simulink model "Bi_DAB"  (R2023a)
settings: Solver=ode23tb  StartTime=0.0  StopTime=0.1  MaxStep=1e-7  RelTol=1e-7
model workspace (MAT data in the model file):
  Ki = 0.0018
  Kp = 0.05
libraries: spsMosfetLib x8, spsSeriesRLCBranchLib x5, spsCurrentMeasurementLib x4, spsVoltageMeasurementLib x4, spsDCVoltageSourceLib x1, spsLinearTransformerLib x1, slpidlib x1, sps_lib x1
settings Model: Creator=gaming3  LastModifiedBy=gaming3

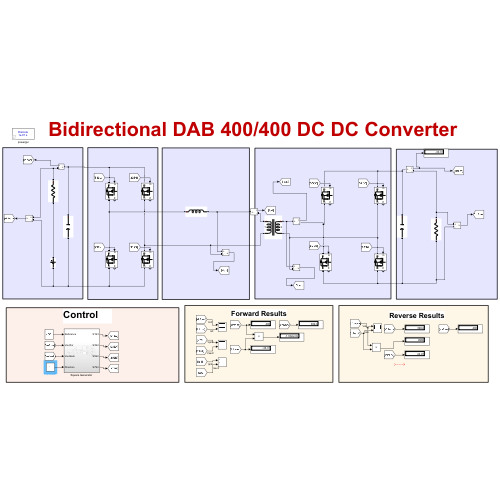
[thumbnail: Simulink's stored preview of the top-level diagram]
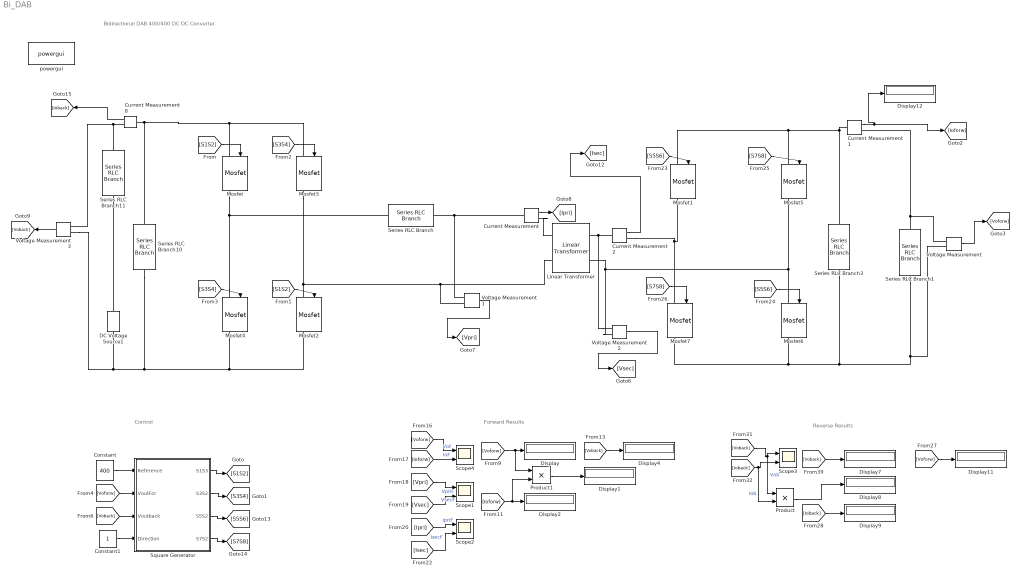
== system Bi_DAB ==
  note: Control
  note: Forward Results
  note: Reverse Results
  note: Bidirectional DAB 400/400 DC DC Converter
  Constant : Constant  Value=400
  Constant1 : Constant
  Current Measurement{,1..2,8} (4 alike) : spsCurrentMeasurementLib/Current Measurement  PhasorSimulation=off  OutputType=Complex  PSBequivalent=0
  DC Voltage Source1 : spsDCVoltageSourceLib/DC Voltage Source  Amplitude=400  Measurements=None
  Display{,1..2,4,7..9,11..12} (9 alike) : Display
  Linear Transformer : spsLinearTransformerLib/Linear Transformer  UNITS=SI  NominalPower=[ 10e3 100e3 ]  winding1=[400 0 0]  winding2=[400 0 0]  ThreeWindings=off  winding3=[3.15e+05 1.9845e+05 12.634]  RmLm=[1.0804e+06 0]  Measurements=None  DataType=on
  Mosfet{,1..7} (8 alike) : spsMosfetLib/Mosfet  Ron=0.1  Lon=0  Rd=0.01  Vfd=0  IC=0  Rs=1e5  Cs=inf  Measurements=on
  Product : Product
  Product1 : Product
  Scope{1..4} (4 alike) : Scope  NumInputPorts=2
  Series RLC Branch : spsSeriesRLCBranchLib/Series RLC Branch  LConnTagsString=__new0  RConnTagsString=__new0  BranchType=L  Resistance=1  Inductance=1.5e-5  SetiL0=off  InitialCurrent=0  Capacitance=1e-6  Setx0=off  InitialVoltage=0  Measurements=None
  Series RLC Branch1 : spsSeriesRLCBranchLib/Series RLC Branch  LConnTagsString=__new0  RConnTagsString=__new0  BranchType=R  Resistance=16  Inductance=1e-3  SetiL0=off  InitialCurrent=0  Capacitance=500e-6  Setx0=on  InitialVoltage=100  Measurements=None
  Series RLC Branch10 : spsSeriesRLCBranchLib/Series RLC Branch  LConnTagsString=__new0  RConnTagsString=__new0  BranchType=C  Resistance=1  Inductance=1e-3  SetiL0=off  InitialCurrent=0  Capacitance=100e-6  Setx0=on  InitialVoltage=400  Measurements=None
  Series RLC Branch11 : spsSeriesRLCBranchLib/Series RLC Branch  LConnTagsString=__new0  RConnTagsString=__new0  BranchType=R  Resistance=0.001  Inductance=1e-3  SetiL0=off  InitialCurrent=0  Capacitance=500e-6  Setx0=on  InitialVoltage=100  Measurements=None
  Series RLC Branch3 : spsSeriesRLCBranchLib/Series RLC Branch  LConnTagsString=__new0  RConnTagsString=__new0  BranchType=C  Resistance=1  Inductance=1e-3  SetiL0=off  InitialCurrent=0  Capacitance=100e-6  Setx0=on  InitialVoltage=400  Measurements=None
  "Square Generator " : Subsystem
  Voltage Measurement{,1..3} (4 alike) : spsVoltageMeasurementLib/Voltage Measurement  PhasorSimulation=off  OutputType=Complex  PSBequivalent=0
  powergui : sps_lib/powergui  Priority=1  SimulationMode=Discrete  SampleTime=1e-07  frequency=60  Iterations=50  frequencyindice=0  Pbase=100e6  ErrMax=1e-4  UnitsV=kV  UnitsW=MW  buscounter=0  FunctionMessages=off  echomessages=off  EnableUseOfTLC=off  CurrentSourceSwitches=off  DisableSnubberDevices=off  DisableRonSwitches=off  DisableVfSwitches=off  DisplayEquations=off  AutomaticDiscreteSolvers=off  SolverType=Tustin/Backward Euler (TBE)  Interpol=off  ExternalGateDelay=off  methode=off  Ts=100  x0status=blocks  SPID=on  SwTol=0  HookPort=off  NonlinearTolerance=1e-4  nMaxIteration=100  ContinueOnMaxIteration=off  RestoreLinks=warning  ResistiveCurrentMeasurement=off  Frange=[0:2:500]  Ylog=off  Xlog=on  ShowGrid=off  save=off  variable=ZData  structure=0  ZoomFFT=off  StartTime=0.0  cycles=1  DisplayStyle=1  fundamental=60  FreqAxis=off  MaxFrequency=1000  frequencyindicesteady=1  RmsSteady=1  display=off
  wires:
  Current Measurement/1 -> [Ipri]
  Current Measurement1/1 -> [Ioforw], Display12/1
  Voltage Measurement1/1 -> [Vpri]
  Current Measurement8/1 -> [Ioback]
  Voltage Measurement3/1 -> [Voback]
  Voltage Measurement2/1 -> [Vsec]
  Current Measurement2/1 -> [Isec]
  "Square Generator "/2(S3S2) -> [S3S4]
  "Square Generator "/4(S7S2) -> [S7S8]
  Constant1/1 -> "Square Generator "/4(Direction)
  "Square Generator "/1(S1S3) -> [S1S2]
  [Voforw] -> "Square Generator "/2(VoutFor)
  Constant/1 -> "Square Generator "/1(Reference)
  "Square Generator "/3(S5S2) -> [S5S6]
  [Ioforw] -> Product1/2, Display2/1
  [Ioforw] -> Scope4/2  "IoF"
  [Isec] -> Scope2/2  "IsecF"
  [Vpri] -> Scope1/1  "VpriF"
  [Voforw] -> Scope4/1  "VoF"
  [Voback] -> Display4/1
  [Voback] -> Display7/1
  [Voforw] -> Display11/1
  [Ipri] -> Scope2/1  "IpriF"
  [Voback] -> Scope3/1, Product/1  "Vob"
  [Voforw] -> Product1/1, Display/1
  [Ioback] -> Display9/1
  Product/1 -> Display8/1
  ? -> ?
  [Ioback] -> Scope3/2, Product/2  "Iob"
  [Vsec] -> Scope1/2  "VsecF"
  [S1S2] -> Mosfet/1
  [S3S4] -> Mosfet3/1
  [S1S2] -> Mosfet2/1
  [S3S4] -> Mosfet4/1
  [S7S8] -> Mosfet7/1
  [S5S6] -> Mosfet6/1
  [S7S8] -> Mosfet5/1
  [S5S6] -> Mosfet1/1
  [Voback] -> "Square Generator "/3(Voutback)
  Voltage Measurement/1 -> [Voforw]
  Product1/1 -> Display1/1
  connections:
  Current Measurement8/RConn1 -- Series RLC Branch11/LConn1 -- Voltage Measurement3/LConn1
  Mosfet1/RConn1 -- Current Measurement2/RConn1 -- Mosfet7/LConn1
  Mosfet5/LConn1 -- Series RLC Branch3/LConn1 -- Current Measurement1/LConn1 -- Mosfet1/LConn1
  Voltage Measurement1/LConn1 -- Current Measurement/LConn1 -- Series RLC Branch/RConn1
  Mosfet3/RConn1 -- Linear Transformer/LConn2 -- Voltage Measurement1/LConn2 -- Mosfet2/LConn1
  Mosfet2/RConn1 -- Series RLC Branch10/RConn1 -- Voltage Measurement3/LConn2 -- DC Voltage Source1/LConn1 -- Mosfet4/RConn1
  Current Measurement8/LConn1 -- Mosfet/LConn1 -- Mosfet3/LConn1 -- Series RLC Branch10/LConn1
  Mosfet5/RConn1 -- Mosfet6/LConn1 -- Linear Transformer/RConn2 -- Voltage Measurement2/LConn2
  Mosfet7/RConn1 -- Series RLC Branch3/RConn1 -- Series RLC Branch1/RConn1 -- Voltage Measurement/LConn2 -- Mosfet6/RConn1
  Voltage Measurement2/LConn1 -- Current Measurement2/LConn1 -- Linear Transformer/RConn1
  Mosfet4/LConn1 -- Series RLC Branch/LConn1 -- Mosfet/RConn1
  Current Measurement/RConn1 -- Linear Transformer/LConn1
  Series RLC Branch1/LConn1 -- Current Measurement1/RConn1 -- Voltage Measurement/LConn1
  Series RLC Branch11/RConn1 -- DC Voltage Source1/RConn1

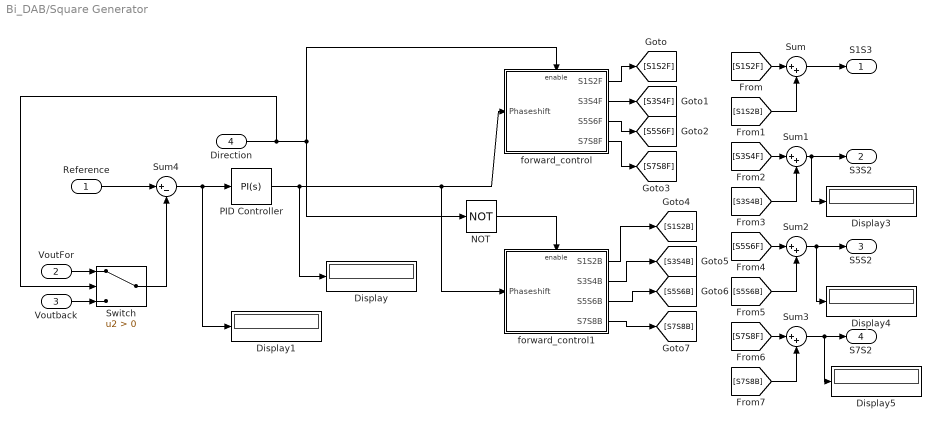
== system Bi_DAB/Square Generator  ==
  Reference : Inport
  VoutFor : Inport  Port=2
  Voutback : Inport  Port=3
  Direction : Inport  Port=4
  Display{,1,3..5} (5 alike) : Display
  NOT : Logic  Operator=NOT  IconShape=distinctive  AllPortsSameDT=off  OutDataTypeStr=boolean
  PID Controller : slpidlib/PID Controller  Controller=PI  Form=Parallel  TimeDomain=Continuous-time  UseExternalTs=off  SampleTime=-1  IntegratorMethod=Forward Euler  FilterMethod=Forward Euler  ControllerParametersSource=internal  P=0.000085  I=0.25  UseKiTs=off  D=0  N=100  UseFilter=on  TunerSelectOption=Transfer Function Based (PID Tuner App)  InitialConditionSource=internal  InitialConditionForIntegrator=0  InitialConditionForFilter=0  DifferentiatorICPrevScaledInput=0  ExternalReset=none  TrackingMode=off  Kt=1  LimitOutput=on  SatLimitsSource=internal  UpperSaturationLimit=0.5  LowerSaturationLimit=-0.5  LinearizeAsGain=on  AntiWindupMode=clamping  Kb=1  LimitIntegrator=off  UpperIntegratorSaturationLimit=inf  LowerIntegratorSaturationLimit=-inf  POutMin=[]  POutMax=[]  IOutMin=[]  IOutMax=[]  DOutMin=[]  DOutMax=[]  NOutMin=[]  NOutMax=[]  SumOutMin=[]  SumOutMax=[]  SaturationOutMin=[]  SaturationOutMax=[]  PParamMin=[]  PParamMax=[]  IParamMin=[]  IParamMax=[]  DParamMin=[]  DParamMax=[]  NParamMin=[]  NParamMax=[]  KbParamMin=[]  KbParamMax=[]  KtParamMin=[]  KtParamMax=[]  KbOutMin=[]  KbOutMax=[]  KtOutMin=[]  KtOutMax=[]  IntegratorOutMin=[]  IntegratorOutMax=[]  FilterOutMin=[]  FilterOutMax=[]  SumI1OutMin=[]  SumI1OutMax=[]  SumI2OutMin=[]  SumI2OutMax=[]  SumI3OutMin=[]  SumI3OutMax=[]  SumI4OutMin=[]  SumI4OutMax=[]  SumDOutMin=[]  SumDOutMax=[]  DifferentiatorOutMin=[]  DifferentiatorOutMax=[]  FilterDiffOutCoefMin=[]  FilterDiffOutCoefMax=[]  ReciprocalOutMin=[]  ReciprocalOutMax=[]  SumDenOutMin=[]  SumDenOutMax=[]  SumNumOutMin=[]  SumNumOutMax=[]  DivideOutMin=[]  DivideOutMax=[]  UdiffTsProdOutMin=[]  UdiffTsProdOutMax=[]  NTsProdOutMin=[]  NTsProdOutMax=[]  UintegralTsProdOutMin=[]  UintegralTsProdOutMax=[]  UngainTsProdOutMin=[]  UngainTsProdOutMax=[]  ClampingZeroOutDataTypeStr=Inherit: Inherit via back propagation  ClampingZeroOutMin=[]  ClampingZeroOutMax=[]  FilterDenConstantOutDataTypeStr=Inherit: Inherit via back propagation  FilterDenConstantOutMin=[]  FilterDenConstantOutMax=[]  PCopyOutDataTypeStr=Inherit: Inherit via back propagation  PCopyOutMin=[]  PCopyOutMax=[]  NCopyOutDataTypeStr=Inherit: Inherit via back propagation  NCopyOutMin=[]  NCopyOutMax=[]  IntegratorContinuousStateAttributes=''  IntegratorStateMustResolveToSignalObject=off  IntegratorRTWStateStorageClass=Auto  FilterContinuousStateAttributes=''  FilterStateMustResolveToSignalObject=off  FilterRTWStateStorageClass=Auto  ParallelPVariant=InternalParameters  IdealPVariant=Disabled  IVariant=InternalParameters  DVariant=Disabled  IntegratorVariant=Continuous  SatVariant=Enabled  AWVariant=ContClampingParallel  PCopyVariant=Disabled  TRVariant=Disabled  FdbkBlocksVariant=Forward  IdealPFdbkVariant=Disabled  SatFdbkVariant=Disabled  DerivativeFilterVariant=Disabled  NVariant=Disabled  NCopyVariant=Disabled_SignalSpec  FilterICVariant=Disabled  IntegratorICVariant=InternalICs  ExternalResetVariant=Disabled  TRSumVariant=Passthrough  SumFdbkVariant=Disabled  SumVariant=Sum_PI  TsampFilterVariant=InternalTs  TsampNgainVariant=Passthrough  TsampIntegralVariant=Disabled_SignalSpec  ExternalSaturationOutDataTypeStr=Inherit: Same as second input
  Sum{,1..3} (4 alike) : Sum  Inputs=|++
  Sum4 : Sum  Inputs=|+-
  Switch : Switch  Criteria=u2 > Threshold  SaturateOnIntegerOverflow=off  InputSameDT=off
  forward_control : Subsystem
  forward_control1 : Subsystem
  S1S3 : Outport
  S3S2 : Outport  Port=2
  S5S2 : Outport  Port=3
  S7S2 : Outport  Port=4
  wires:
  forward_control/1(S1S2F) -> [S1S2F]
  forward_control/2(S3S4F) -> [S3S4F]
  forward_control/3(S5S6F) -> [S5S6F]
  forward_control/4(S7S8F) -> [S7S8F]
  [S1S2F] -> Sum/1
  [S1S2B] -> Sum/2
  [S3S4B] -> Sum1/2
  [S3S4F] -> Sum1/1
  [S7S8F] -> Sum3/1
  [S7S8B] -> Sum3/2
  [S5S6B] -> Sum2/2
  [S5S6F] -> Sum2/1
  Sum/1 -> S1S3/1
  Sum1/1 -> Display3/1, S3S2/1
  Sum2/1 -> Display4/1, S5S2/1
  Sum3/1 -> Display5/1, S7S2/1
  Direction/1 -> Switch/2, forward_control/Enable, NOT/1
  Reference/1 -> Sum4/1
  Sum4/1 -> Display1/1, PID Controller/1
  PID Controller/1 -> Display/1, forward_control1/1(Phaseshift), forward_control/1(Phaseshift)
  forward_control1/1(S1S2B) -> [S1S2B]
  forward_control1/2(S3S4B) -> [S3S4B]
  forward_control1/3(S5S6B) -> [S5S6B]
  forward_control1/4(S7S8B) -> [S7S8B]
  NOT/1 -> forward_control1/Enable
  Switch/1 -> Sum4/2
  VoutFor/1 -> Switch/1
  Voutback/1 -> Switch/3

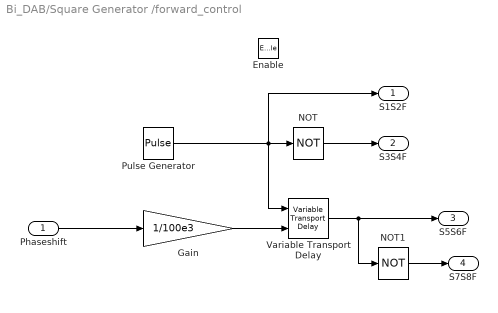
== system Bi_DAB/Square Generator /forward_control ==
  Phaseshift : Inport
  Enable : EnablePort
  Gain : Gain  Gain=1/100e3
  NOT : Logic  Operator=NOT  AllPortsSameDT=off  OutDataTypeStr=boolean
  NOT1 : Logic  Operator=NOT  AllPortsSameDT=off  OutDataTypeStr=boolean
  Pulse Generator : DiscretePulseGenerator  PulseType=Time based  Period=1/100e3  PulseWidth=50
  Variable Transport Delay : VariableTransportDelay  MaximumDelay=10
  S1S2F : Outport
  S3S4F : Outport  Port=2
  S5S6F : Outport  Port=3
  S7S8F : Outport  Port=4
  wires:
  Pulse Generator/1 -> Variable Transport Delay/1, S1S2F/1, NOT/1
  NOT/1 -> S3S4F/1
  Gain/1 -> Variable Transport Delay/2
  Variable Transport Delay/1 -> NOT1/1, S5S6F/1
  NOT1/1 -> S7S8F/1
  Phaseshift/1 -> Gain/1

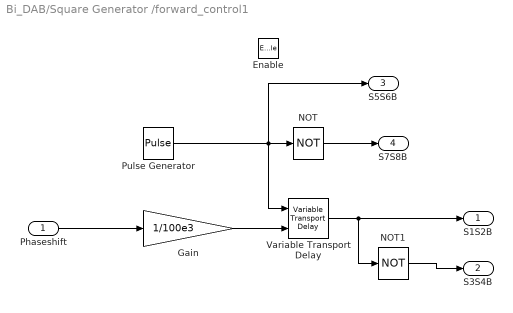
== system Bi_DAB/Square Generator /forward_control1 ==
  Phaseshift : Inport
  Enable : EnablePort
  Gain : Gain  Gain=1/100e3
  NOT : Logic  Operator=NOT  AllPortsSameDT=off  OutDataTypeStr=boolean
  NOT1 : Logic  Operator=NOT  AllPortsSameDT=off  OutDataTypeStr=boolean
  Pulse Generator : DiscretePulseGenerator  PulseType=Time based  Period=1/100e3  PulseWidth=50
  Variable Transport Delay : VariableTransportDelay  MaximumDelay=10
  S1S2B : Outport
  S3S4B : Outport  Port=2
  S5S6B : Outport  Port=3
  S7S8B : Outport  Port=4
  wires:
  Phaseshift/1 -> Gain/1
  Variable Transport Delay/1 -> S1S2B/1, NOT1/1
  Gain/1 -> Variable Transport Delay/2
  Pulse Generator/1 -> S5S6B/1, NOT/1, Variable Transport Delay/1
  NOT1/1 -> S3S4B/1
  NOT/1 -> S7S8B/1
